simulink model "GUI_Inv_Android"  (R2022b)
settings: Solver=FixedStepAuto  StartTime=0.0  StopTime=inf  RelTol=1e-3
InitFcn:
  | samplerate_udp = 100e-3;
  | PWMclock = 100e6;
libraries: androiduilib x21, simulink x4, androidcommunicationlib x2
settings Model: Creator=The MathWorks, Inc.  LastModifiedBy=ReiterTo
settings SolverCC: AlgebraicLoopSolver=TrustRegion
settings DataIOCC: ReturnWorkspaceOutputs=off
settings OptimizationCC: PassReuseOutputArgsThreshold=0  MaxStackSize=64
settings DebuggingCC: ParameterPrecisionLossMsg=none  ParameterTunabilityLossMsg=error  UnconnectedInputMsg=warning  UnconnectedOutputMsg=warning  UnconnectedLineMsg=warning  SFMachineParentedDataDiag=warning  ArithmeticOperatorsInVariantConditions=warning
settings HardwareCC: ProdBitPerPointer=32  ProdBitPerSizeT=32  ProdBitPerPtrDiffT=32  ProdLargestAtomicInteger=Long  ProdLargestAtomicFloat=Double  ProdWordSize=32  ProdHWDeviceType=ARM Compatible->ARM Cortex  UseEmbeddedCoderFeatures=off  UseSimulinkCoderFeatures=off
settings ModelReferenceCC: EnableRefExpFcnMdlSchedulingChecks=on
settings SFSimCC: SimUseLocalCustomCode=off  CustomCodeUndefinedFunction=UseInterfaceOnly
settings RTWCC: Description=Embedded Coder  SystemTargetFile=ert.tlc  HardwareBoard=Android Device  TLCOptions="-aInlineSetEventsForThisBaseRateFcn=TLC_FALSE -aSuppressMultiTaskScheduler=TLC_FALSE  -aRateBasedStepFcn=0"  TemplateMakefile=ert_default_tmf  GenerateReport=on  RTWUseLocalCustomCode=off  Toolchain=Android SDK/NDK Tools  LaunchReport=on
settings CodeAppCC: ForceParamTrailComments=on  OperatorAnnotations=on  StateflowObjectComments=on  MATLABSourceComments=on
settings ERTTargetCC: ERTCustomFileBanners=off  SupportContinuousTime=on  SupportNonInlinedSFcns=on  RemoveResetFunc=off  ModelStepFunctionPrototypeControlCompliant=off

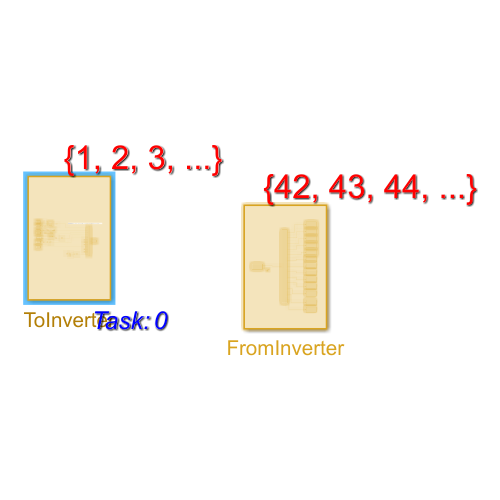
[thumbnail: Simulink's stored preview of the top-level diagram]
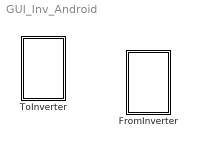
== system GUI_Inv_Android ==
  FromInverter : Subsystem
  ToInverter : Subsystem  Priority=0

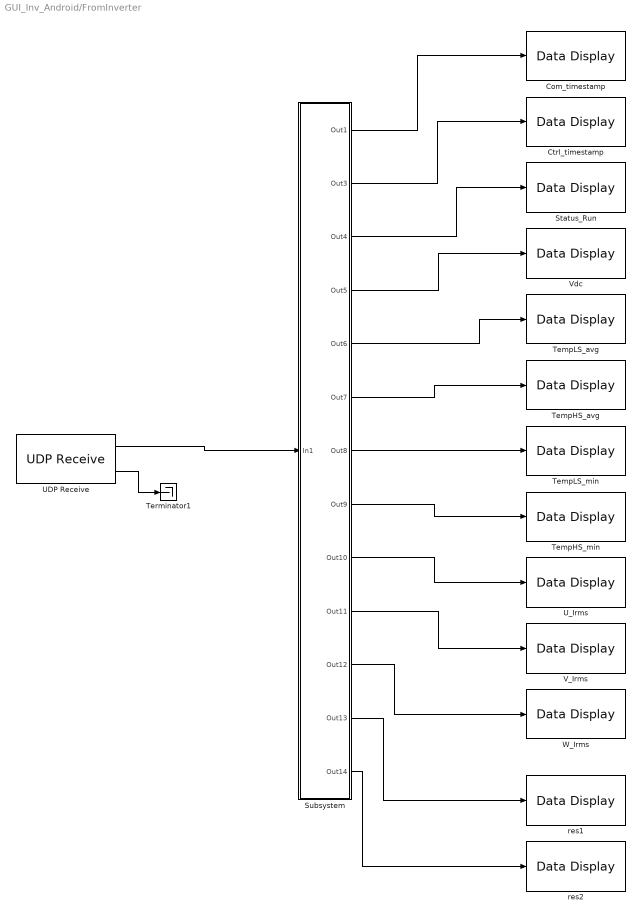
== system GUI_Inv_Android/FromInverter ==
  Com_timestamp : androiduilib/Data Display  Priority=10  DataDisplayId=GUI_Inv_Android/FromInverter/Com_timestamp  Format=Integer  Precision=6  SimulateUsing=Code generation  blockPlatform=Android
  Ctrl_timestamp : androiduilib/Data Display  Priority=20  DataDisplayId=GUI_Inv_Android/FromInverter/Ctrl_timestamp  Format=Integer  Precision=6  SimulateUsing=Code generation  blockPlatform=Android
  Status_Run : androiduilib/Data Display  Priority=30  DataDisplayId=GUI_Inv_Android/FromInverter/Status_Run  Format=Integer  Precision=6  SimulateUsing=Code generation  blockPlatform=Android
  Subsystem : Subsystem
  TempHS_avg : androiduilib/Data Display  Priority=60  DataDisplayId=GUI_Inv_Android/FromInverter/TempHS_avg  Format=Integer  Precision=6  SimulateUsing=Code generation  blockPlatform=Android
  TempHS_min : androiduilib/Data Display  Priority=80  DataDisplayId=GUI_Inv_Android/FromInverter/TempHS_min  Format=Integer  Precision=6  SimulateUsing=Code generation  blockPlatform=Android
  TempLS_avg : androiduilib/Data Display  Priority=50  DataDisplayId=GUI_Inv_Android/FromInverter/TempLS_avg  Format=Integer  Precision=6  SimulateUsing=Code generation  blockPlatform=Android
  TempLS_min : androiduilib/Data Display  Priority=70  DataDisplayId=GUI_Inv_Android/FromInverter/TempLS_min  Format=Integer  Precision=6  SimulateUsing=Code generation  blockPlatform=Android
  Terminator1 : Terminator
  UDP Receive : androidcommunicationlib/UDP Receive  localURL='0.0.0.0'  localPort=60000  remoteURL='0.0.0.0'  remotePort=-1  recvBufferSize=8192  signalDatatype=uint16  dims=15  isVarSize=off  showBlockingTime=off  blockingTime=0  sampletime=samplerate_udp  blockPlatform=Android
  U_Irms : androiduilib/Data Display  Priority=90  DataDisplayId=GUI_Inv_Android/FromInverter/U_Irms  Format=Integer  Precision=6  SimulateUsing=Code generation  blockPlatform=Android
  V_Irms : androiduilib/Data Display  Priority=100  DataDisplayId=GUI_Inv_Android/FromInverter/V_Irms  Format=Integer  Precision=6  SimulateUsing=Code generation  blockPlatform=Android
  Vdc : androiduilib/Data Display  Priority=40  DataDisplayId=GUI_Inv_Android/FromInverter/Vdc  Format=Integer  Precision=6  SimulateUsing=Code generation  blockPlatform=Android
  W_Irms : androiduilib/Data Display  Priority=110  DataDisplayId=GUI_Inv_Android/FromInverter/W_Irms  Format=Integer  Precision=6  SimulateUsing=Code generation  blockPlatform=Android
  res1 : androiduilib/Data Display  Priority=120  DataDisplayId=GUI_Inv_Android/FromInverter/res1  Format=Integer  Precision=6  SimulateUsing=Code generation  blockPlatform=Android
  res2 : androiduilib/Data Display  Priority=130  DataDisplayId=GUI_Inv_Android/FromInverter/res2  Format=Integer  Precision=6  SimulateUsing=Code generation  blockPlatform=Android
  wires:
  Subsystem/1(Out1) -> Com_timestamp/1
  UDP Receive/1 -> Subsystem/1(In1)
  UDP Receive/2 -> Terminator1/1
  Subsystem/2(Out3) -> Ctrl_timestamp/1
  Subsystem/3(Out4) -> Status_Run/1
  Subsystem/4(Out5) -> Vdc/1
  Subsystem/5(Out6) -> TempLS_avg/1
  Subsystem/6(Out7) -> TempHS_avg/1
  Subsystem/7(Out8) -> TempLS_min/1
  Subsystem/8(Out9) -> TempHS_min/1
  Subsystem/9(Out10) -> U_Irms/1
  Subsystem/10(Out11) -> V_Irms/1
  Subsystem/11(Out12) -> W_Irms/1
  Subsystem/12(Out13) -> res1/1
  Subsystem/13(Out14) -> res2/1

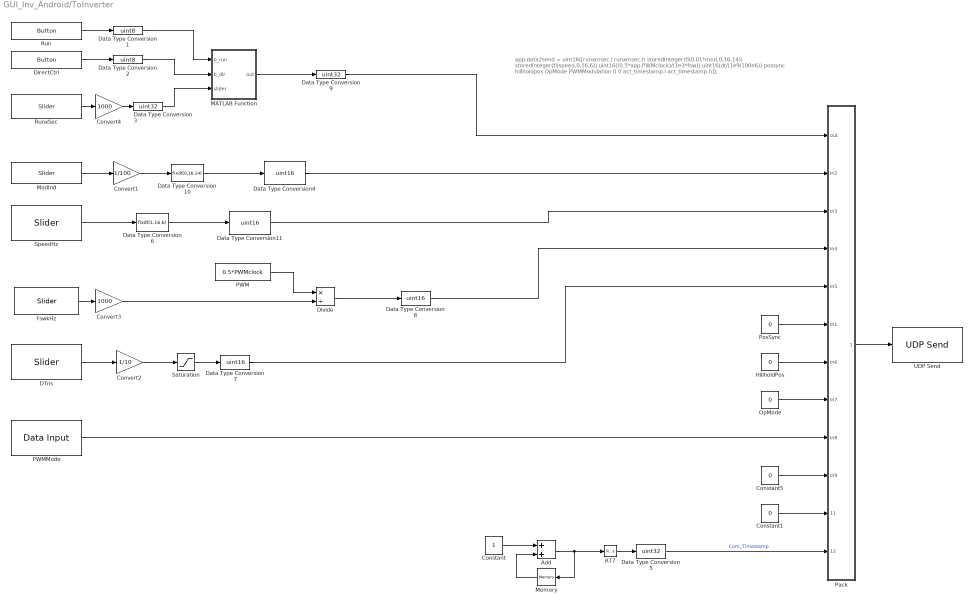
== system GUI_Inv_Android/ToInverter ==
  note: app.data2send = uint16([runxmsec.l runxmsec.h storedInteger(fi(0.01*mod,0,16,14)) storedInteger(fi(speed,0,16,6)) uint16((0.5*app.PWMclock)/(1e3*fsw)) uint16(dt/(1e9/100e6)) possync hillholdpos OpMode PWMModulation 0 0 act_timestamp.l act_timestamp.h]);
  Add : Sum
  Constant : Constant  OutDataTypeStr=uint32  SampleTime=samplerate_udp
  Constant1 : Constant  Value=0  OutDataTypeStr=uint16  SampleTime=samplerate_udp
  Constant5 : Constant  Value=0  OutDataTypeStr=uint16  SampleTime=samplerate_udp
  Convert1 : Gain  Gain=1/100  OutDataTypeStr=single
  Convert2 : Gain  Gain=1/10  OutDataTypeStr=single
  Convert3 : Gain  Gain=1000  OutDataTypeStr=single
  Convert4 : Gain  Gain=1000  OutDataTypeStr=single
  DTns : androiduilib/Slider  Min=0  Value=500  Max=2500  Resolution=50  SliderId=GUI_Inv_Android/ToInverter/DTns  SampleTime=samplerate_udp  BlockPlatform=Android
  Data Type Conversion1 : DataTypeConversion  OutDataTypeStr=uint8  RndMeth=Simplest  SaturateOnIntegerOverflow=off
  Data Type Conversion10 : DataTypeConversion  OutDataTypeStr=fixdt(0,16,14)  RndMeth=Simplest  SaturateOnIntegerOverflow=off  LockScale=on
  Data Type Conversion11 : DataTypeConversion  OutDataTypeStr=uint16  ConvertRealWorld=Stored Integer (SI)  RndMeth=Simplest  SaturateOnIntegerOverflow=off
  Data Type Conversion2 : DataTypeConversion  OutDataTypeStr=uint8  RndMeth=Simplest  SaturateOnIntegerOverflow=off
  Data Type Conversion3 : DataTypeConversion  OutDataTypeStr=uint32  RndMeth=Simplest  SaturateOnIntegerOverflow=off
  Data Type Conversion4 : DataTypeConversion  OutDataTypeStr=uint16  ConvertRealWorld=Stored Integer (SI)  RndMeth=Simplest  SaturateOnIntegerOverflow=off
  Data Type Conversion5 : DataTypeConversion  OutDataTypeStr=uint32  SaturateOnIntegerOverflow=off  RndMeth=Floor
  Data Type Conversion6 : DataTypeConversion  OutDataTypeStr=fixdt(1,16,6)  RndMeth=Simplest  SaturateOnIntegerOverflow=off  LockScale=on
  Data Type Conversion7 : DataTypeConversion  OutDataTypeStr=uint16  SaturateOnIntegerOverflow=off  RndMeth=Floor
  Data Type Conversion8 : DataTypeConversion  OutDataTypeStr=uint16  SaturateOnIntegerOverflow=off  RndMeth=Floor
  Data Type Conversion9 : DataTypeConversion  OutDataTypeStr=uint32  RndMeth=Simplest  SaturateOnIntegerOverflow=off
  DirectCtrl : androiduilib/Button  ButtonState=Not pressed  ButtonId=GUI_Inv_Android/ToInverter/DirectCtrl  State=off  SampleTime=samplerate_udp  BlockPlatform=Android
  Divide : Product  Inputs=*/  OutDataTypeStr=single  RndMeth=Simplest
  FswkHz : androiduilib/Slider  Min=2  Value=10  Max=60  Resolution=0.5  SliderId=GUI_Inv_Android/ToInverter/FswkHz  SampleTime=samplerate_udp  BlockPlatform=Android
  HillholdPos : Constant  Value=0  OutDataTypeStr=uint16  SampleTime=samplerate_udp
  MATLAB Function : MATLAB Function  TreatAsAtomicUnit=on
  Memory : Memory  InheritSampleTime=on  LinearizeMemory=on  StateName=ctrl_timestamp_z1
  ModInd : androiduilib/Slider  Min=0  Value=1  Max=100  Resolution=0.5  SliderId=GUI_Inv_Android/ToInverter/ModInd  SampleTime=samplerate_udp  BlockPlatform=Android
  OpMode : Constant  Value=0  OutDataTypeStr=uint16  SampleTime=samplerate_udp
  PWM : Constant  Value=0.5*PWMclock  OutDataTypeStr=single  SampleTime=samplerate_udp
  PWMMode : androiduilib/Data Input  isCharVector=off  Value=0  CharVector=Hello World  OutputDataType=uint16  maxCharVectorSize=100  DataInputId=GUI_Inv_Android/ToInverter/PWMMode  SampleTime=0.1
  Pack : Subsystem
  PosSync : Constant  Value=0  OutDataTypeStr=uint16  SampleTime=samplerate_udp
  RT7 : RateTransition  Deterministic=off  OutPortSampleTime=samplerate_udp
  Run : androiduilib/Button  ButtonState=Not pressed  ButtonId=GUI_Inv_Android/ToInverter/Run  State=off  SampleTime=samplerate_udp  BlockPlatform=Android
  RunxSec : androiduilib/Slider  Min=1  Value=10  Max=60  Resolution=1  SliderId=GUI_Inv_Android/ToInverter/RunxSec  SampleTime=samplerate_udp  BlockPlatform=Android
  Saturation : Saturate  UpperLimit=255  LowerLimit=0  RndMeth=Simplest
  SpeedHz : androiduilib/Slider  Min=0  Value=100  Max=600  Resolution=10  SliderId=GUI_Inv_Android/ToInverter/SpeedHz  SampleTime=samplerate_udp  BlockPlatform=Android
  UDP Send : androidcommunicationlib/UDP Send  remoteURL='255.255.255.255'  remotePort=50000  localURL='0.0.0.0'  localPortSource=Automatically determine  localPort=-1  sampletime=-1  blockPlatform=Android  separateLengthPort=0
  wires:
  Data Type Conversion2/1 -> MATLAB Function/2(b_dir)
  HillholdPos/1 -> Pack/7(In6)
  Run/1 -> Data Type Conversion1/1
  Constant/1 -> Add/1
  RunxSec/1 -> Convert4/1
  DirectCtrl/1 -> Data Type Conversion2/1
  Add/1 -> RT7/1, Memory/1
  Data Type Conversion8/1 -> Pack/4(In4)
  Data Type Conversion1/1 -> MATLAB Function/1(b_run)
  Data Type Conversion3/1 -> MATLAB Function/3(slider)
  DTns/1 -> Convert2/1
  ModInd/1 -> Convert1/1
  Data Type Conversion4/1 -> Pack/2(In2)
  MATLAB Function/1(out) -> Data Type Conversion9/1
  PosSync/1 -> Pack/6(In1)
  Convert1/1 -> Data Type Conversion10/1
  Memory/1 -> Add/2
  Data Type Conversion9/1 -> Pack/1(out)
  RT7/1 -> Data Type Conversion5/1
  Pack/1(Out1) -> UDP Send/1
  FswkHz/1 -> Convert3/1
  PWM/1 -> Divide/1
  Divide/1 -> Data Type Conversion8/1
  Convert3/1 -> Divide/2
  Convert4/1 -> Data Type Conversion3/1
  SpeedHz/1 -> Data Type Conversion6/1
  Data Type Conversion10/1 -> Data Type Conversion4/1
  Data Type Conversion6/1 -> Data Type Conversion11/1
  Data Type Conversion11/1 -> Pack/3(In3)
  Convert2/1 -> Saturation/1
  Saturation/1 -> Data Type Conversion7/1
  Data Type Conversion7/1 -> Pack/5(In5)
  OpMode/1 -> Pack/8(In7)
  PWMMode/1 -> Pack/9(In8)
  Constant5/1 -> Pack/10(In9)
  Data Type Conversion5/1 -> Pack/12(Com_Timestamp)  "Com_Timestamp"
  Constant1/1 -> Pack/11(In10)

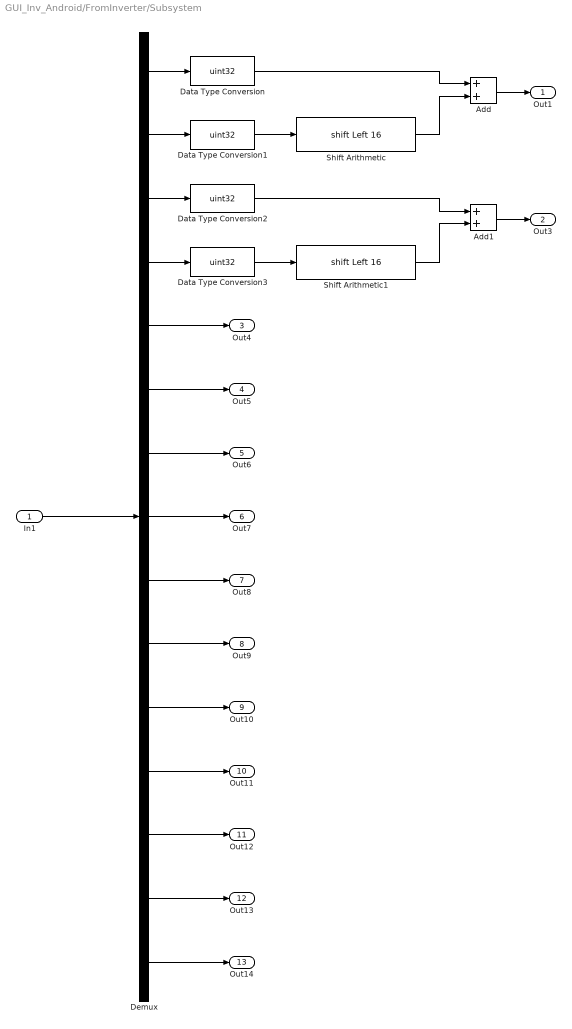
== system GUI_Inv_Android/FromInverter/Subsystem ==
  In1 : Inport
  Add : Sum
  Add1 : Sum
  Data Type Conversion{,1..3} (4 alike) : DataTypeConversion  OutDataTypeStr=uint32  SaturateOnIntegerOverflow=off  RndMeth=Floor
  Demux : Demux  Outputs=15
  Shift Arithmetic : ArithShift  BitShiftNumber=16  BitShiftDirection=Left
  Shift Arithmetic1 : ArithShift  BitShiftNumber=16  BitShiftDirection=Left
  Out1 : Outport
  Out3 : Outport  Port=2
  Out4 : Outport  Port=3
  Out5 : Outport  Port=4
  Out6 : Outport  Port=5
  Out7 : Outport  Port=6
  Out8 : Outport  Port=7
  Out9 : Outport  Port=8
  Out10 : Outport  Port=9
  Out11 : Outport  Port=10
  Out12 : Outport  Port=11
  Out13 : Outport  Port=12
  Out14 : Outport  Port=13
  wires:
  In1/1 -> Demux/1
  Demux/6 -> Out5/1
  Demux/5 -> Out4/1
  Demux/3 -> Data Type Conversion2/1
  Demux/1 -> Data Type Conversion/1
  Demux/2 -> Data Type Conversion1/1
  Data Type Conversion1/1 -> Shift Arithmetic/1
  Data Type Conversion/1 -> Add/1
  Shift Arithmetic/1 -> Add/2
  Add/1 -> Out1/1
  Demux/7 -> Out6/1
  Demux/8 -> Out7/1
  Demux/9 -> Out8/1
  Demux/10 -> Out9/1
  Demux/11 -> Out10/1
  Demux/12 -> Out11/1
  Demux/13 -> Out12/1
  Demux/14 -> Out13/1
  Demux/15 -> Out14/1
  Add1/1 -> Out3/1
  Data Type Conversion2/1 -> Add1/1
  Shift Arithmetic1/1 -> Add1/2
  Data Type Conversion3/1 -> Shift Arithmetic1/1
  Demux/4 -> Data Type Conversion3/1

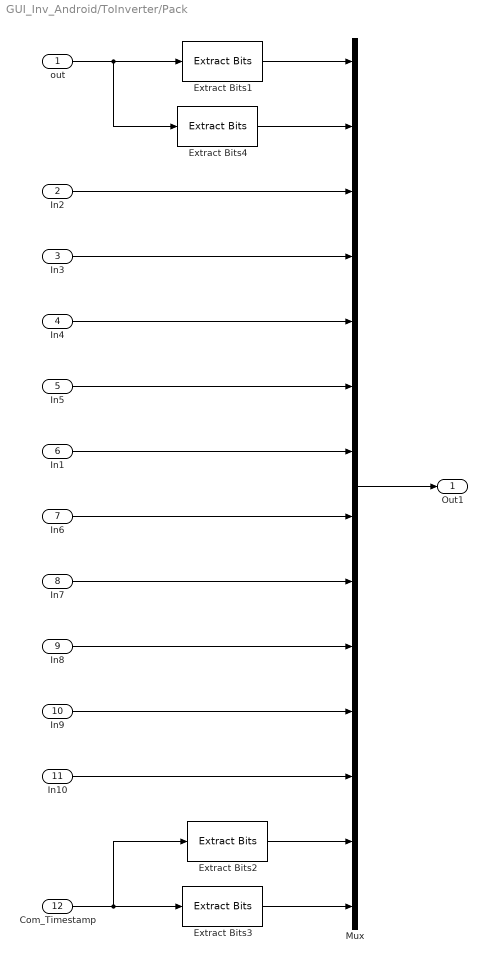
== system GUI_Inv_Android/ToInverter/Pack ==
  out : Inport
  In2 : Inport  Port=2
  In3 : Inport  Port=3
  In4 : Inport  Port=4
  In5 : Inport  Port=5
  In1 : Inport  Port=6
  In6 : Inport  Port=7
  In7 : Inport  Port=8
  In8 : Inport  Port=9
  In9 : Inport  Port=10
  In10 : Inport  Port=11
  Com_Timestamp : Inport  Port=12
  Extract Bits1 : simulink/Logic and Bit Operations/Extract Bits  bitsToExtract=Lower half  numBits=8  bitIdxRange=[0 7]  outScalingMode=Treat bit field as an integer
  Extract Bits2 : simulink/Logic and Bit Operations/Extract Bits  bitsToExtract=Lower half  numBits=8  bitIdxRange=[0 7]  outScalingMode=Treat bit field as an integer
  Extract Bits3 : simulink/Logic and Bit Operations/Extract Bits  bitsToExtract=Upper half  numBits=8  bitIdxRange=[0 7]  outScalingMode=Treat bit field as an integer
  Extract Bits4 : simulink/Logic and Bit Operations/Extract Bits  bitsToExtract=Upper half  numBits=8  bitIdxRange=[0 7]  outScalingMode=Treat bit field as an integer
  Mux : Mux  Inputs=14
  Out1 : Outport
  wires:
  Mux/1 -> Out1/1
  Extract Bits1/1 -> Mux/1
  Extract Bits4/1 -> Mux/2
  In4/1 -> Mux/5
  In5/1 -> Mux/6
  In3/1 -> Mux/4
  In2/1 -> Mux/3
  out/1 -> Extract Bits4/1, Extract Bits1/1
  In1/1 -> Mux/7
  In6/1 -> Mux/8
  In7/1 -> Mux/9
  In8/1 -> Mux/10
  In9/1 -> Mux/11
  In10/1 -> Mux/12
  Extract Bits2/1 -> Mux/13
  Extract Bits3/1 -> Mux/14
  Com_Timestamp/1 -> Extract Bits2/1, Extract Bits3/1

== matlab function GUI_Inv_Android/ToInverter/MATLAB Function ==
  data: out output; b_run input; b_dir input; slider input
function out  = fcn(b_run,b_dir,slider)

if (b_run == 0)
    out = uint32(0);
else
    if (b_dir == 0)
        out = uint32(slider);
    else
        out = uint32(hex2dec('0xFFFFFFFF'));
    end
end
